simulink model "ElectronicGate"  (R2022b)
settings: Solver=VariableStepAuto  StartTime=0.0  StopTime=10.0  RelTol=1e-3
settings Model: Creator=chiar  LastModifiedBy=chiar
settings OptimizationCC: DefaultParameterBehavior=Inlined  UseDivisionForNetSlopeComputation=on  GainParamInheritBuiltInType=on  UseFloatMulNetSlope=on  InlineInvariantSignals=on  PassReuseOutputArgsAs=Individual arguments  ZeroExternalMemoryAtStartup=off  ZeroInternalMemoryAtStartup=off  NoFixptDivByZeroProtection=on  EfficientFloat2IntCast=on  LifeSpan=1  OptimizeBlockOrder=speed  DifferentSizesBufferReuse=on  EfficientTunableParamExpr=on
settings DebuggingCC: ParameterTunabilityLossMsg=error
settings HardwareCC: ProdBitPerPointer=32  ProdBitPerSizeT=32  ProdBitPerPtrDiffT=32  ProdLargestAtomicInteger=Long  ProdLargestAtomicFloat=Double  ProdWordSize=32  ProdLongLongMode=on  ProdHWDeviceType=ARM Compatible->ARM Cortex-M
settings SFSimCC: MATLABDynamicMemAlloc=off
settings RTWCC: Description=Embedded Coder  SystemTargetFile=ert.tlc  TemplateMakefile=ert_default_tmf
settings CodeAppCC: ForceParamTrailComments=on  IgnoreCustomStorageClasses=off  OperatorAnnotations=on  SimulinkDataObjDesc=on  SFDataObjDesc=on  CustomSymbolStrGlobalVar=rt$N$M  CustomSymbolStrType=$N$M  CustomSymbolStrFcn=$N$M$F  CustomSymbolStrMacro=$N$M  InsertBlockDesc=on
settings ERTTargetCC: TargetLangStandard=C99 (ISO)  GenerateSampleERTMain=on  IncludeMdlTerminateFcn=off  CombineSignalStateStructs=on  SupportComplex=off  SupportContinuousTime=on  SupportNonInlinedSFcns=on  InlinedParameterPlacement=NonHierarchical  ERTCustomFileTemplate=example_file_process.tlc  ERTFilePackagingFormat=CompactWithDataFile
settings ConfigComp: CovEnable=on  RecordCoverage=on  CovHTMLOptions=-sRT=1 -sVT=0 -aTS=1 -agT=1 -bRG=1 -bTC=1 -hTR=0 -nFC=0 -nFD=1 -scm=1 -bcm=1 -xEv=0 -xEM=0 -req=1  CovCumulativeReport=on  CovModelRefEnable=on

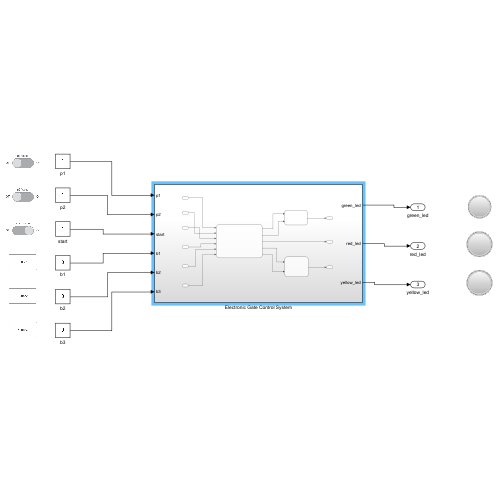
[thumbnail: Simulink's stored preview of the top-level diagram]
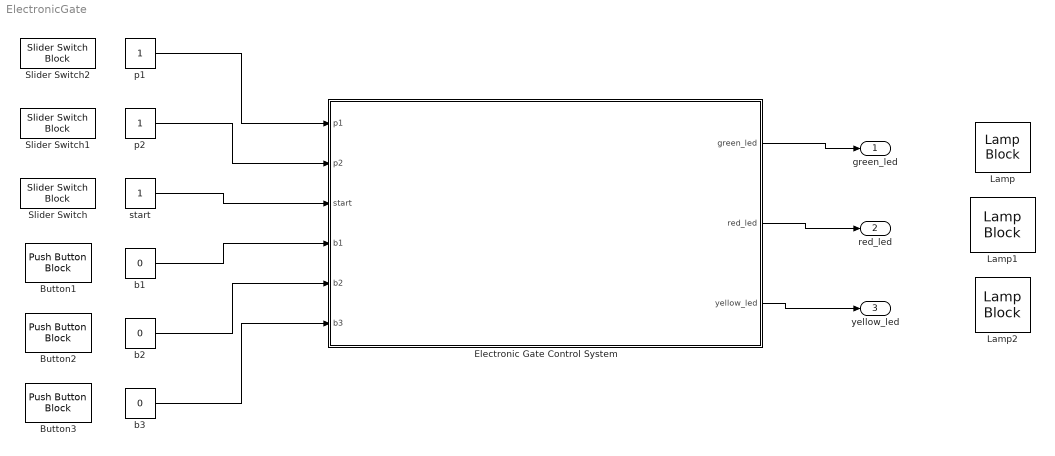
== system ElectronicGate ==
  Button1 : PushButtonBlock  ButtonText=Button1  ButtonType=Latch  OffValue=0.000000
  Button2 : PushButtonBlock  ButtonText=Button2  ButtonType=Latch  OffValue=0.000000
  Button3 : PushButtonBlock  ButtonText=Button3  ButtonType=Latch  OffValue=0.000000
  Electronic Gate Control System : Subsystem
  Lamp : LampBlock  LabelPosition=Hide
  Lamp1 : LampBlock  LabelPosition=Hide
  Lamp2 : LampBlock  LabelPosition=Hide
  Slider Switch : SliderSwitchBlock
      settings: Values={{'Off', 'On'}, [0 1]}
  Slider Switch1 : SliderSwitchBlock
      settings: Values={{'Off', 'On'}, [1 0]}
  Slider Switch2 : SliderSwitchBlock
      settings: Values={{'Off', 'On'}, [1 0]}
  b1 : Constant  Value=0  OutDataTypeStr=boolean
  b2 : Constant  Value=0  OutDataTypeStr=boolean
  b3 : Constant  Value=0  OutDataTypeStr=boolean
  p1 : Constant  OutDataTypeStr=boolean
  p2 : Constant  OutDataTypeStr=boolean
  start : Constant  OutDataTypeStr=boolean
  green_led : Outport  OutDataTypeStr=boolean
  red_led : Outport  Port=2  OutDataTypeStr=boolean
  yellow_led : Outport  Port=3  OutDataTypeStr=boolean
  wires:
  Electronic Gate Control System/1(green_led) -> green_led/1
  Electronic Gate Control System/2(red_led) -> red_led/1
  Electronic Gate Control System/3(yellow_led) -> yellow_led/1
  p1/1 -> Electronic Gate Control System/1(p1)
  p2/1 -> Electronic Gate Control System/2(p2)
  start/1 -> Electronic Gate Control System/3(start)
  b1/1 -> Electronic Gate Control System/4(b1)
  b2/1 -> Electronic Gate Control System/5(b2)
  b3/1 -> Electronic Gate Control System/6(b3)

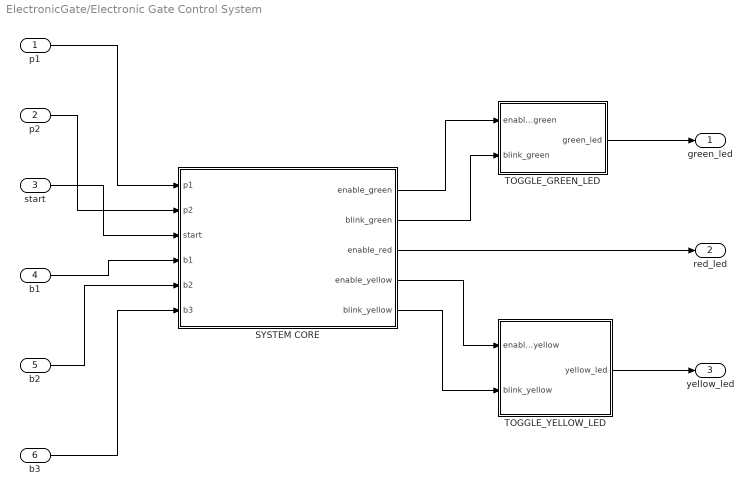
== system ElectronicGate/Electronic Gate Control System ==
  p1 : Inport  OutDataTypeStr=boolean
  p2 : Inport  Port=2  OutDataTypeStr=boolean
  start : Inport  Port=3  OutDataTypeStr=boolean
  b1 : Inport  Port=4  OutDataTypeStr=boolean
  b2 : Inport  Port=5  OutDataTypeStr=boolean
  b3 : Inport  Port=6  OutDataTypeStr=boolean
  SYSTEM CORE : Stateflow chart  TreatAsAtomicUnit=on
  TOGGLE_GREEN_LED : Stateflow chart  TreatAsAtomicUnit=on
  TOGGLE_YELLOW_LED : Stateflow chart  TreatAsAtomicUnit=on
  green_led : Outport  OutDataTypeStr=boolean
  red_led : Outport  Port=2  OutDataTypeStr=boolean
  yellow_led : Outport  Port=3  OutDataTypeStr=boolean
  wires:
  SYSTEM CORE/4(enable_yellow) -> TOGGLE_YELLOW_LED/1(enable_yellow)
  TOGGLE_YELLOW_LED/1(yellow_led) -> yellow_led/1
  p2/1 -> SYSTEM CORE/2(p2)
  start/1 -> SYSTEM CORE/3(start)
  SYSTEM CORE/5(blink_yellow) -> TOGGLE_YELLOW_LED/2(blink_yellow)
  p1/1 -> SYSTEM CORE/1(p1)
  SYSTEM CORE/1(enable_green) -> TOGGLE_GREEN_LED/1(enable_green)
  b3/1 -> SYSTEM CORE/6(b3)
  SYSTEM CORE/2(blink_green) -> TOGGLE_GREEN_LED/2(blink_green)
  b2/1 -> SYSTEM CORE/5(b2)
  SYSTEM CORE/3(enable_red) -> red_led/1
  TOGGLE_GREEN_LED/1(green_led) -> green_led/1
  b1/1 -> SYSTEM CORE/4(b1)

== stateflow chart ElectronicGate/Electronic Gate Control System/TOGGLE_GREEN_LED ==
  state TOGGLE_GREEN
    state SWITCH
      state SWITCH_OFF
        en: green_led = OFF
      state SWITCH_ON
        en: green_led = ON
      (default) -> SWITCH_OFF
      SWITCH_OFF -> SWITCH_ON : [enable_green == ON]
      SWITCH_ON -> SWITCH_OFF : [enable_green == OFF]
    state BLINKING
      state BLINKING_ON
        en: green_led = ON
      state BLINKING_OFF
        en: green_led = OFF
      (default) -> BLINKING_ON
      BLINKING_OFF -> BLINKING_ON : [after(TGREEN, sec)]
      BLINKING_ON -> BLINKING_OFF : [after(TGREEN, sec)]
    (default) -> SWITCH
    SWITCH -> BLINKING : [blink_green == ON]
    BLINKING -> SWITCH : [blink_green == OFF]
  data: TGREEN constant double =1; OFF constant boolean =0; ON constant boolean =1; enable_green input boolean; green_led output boolean; blink_green input boolean

== stateflow chart ElectronicGate/Electronic Gate Control System/SYSTEM CORE ==
  state SYSTEM
    state GATE [parallel]
      settings: executionOrder=3
      state INACTIVE
        en:
        enable_green = OFF;
        enable_yellow = OFF;
        enable_red = OFF;
        blink_green = OFF;
        blink_yellow = OFF;
      state ACTIVE
        state IS_OPENING
          en:
          enable_red = OFF;
          enable_yellow=OFF;
          enable_green=OFF;
          blink_green = OFF;
          blink_yellow = ON;
        state OPEN
          state GREEN_BLK_OFF
            en:
            enable_green = ON;
            enable_red = ON;
            enable_yellow = ON;
            blink_green = OFF;
            blink_yellow = OFF;
          state GREEN_BLK_ON
            en:
            enable_green = OFF;
            enable_red = OFF;
            enable_yellow = OFF;
            blink_green = ON;
            blink_yellow = OFF;
          (default) -> SYSTEM.GATE.ACTIVE.OPEN.GREEN_BLK_OFF
          SYSTEM.GATE.ACTIVE.OPEN.GREEN_BLK_ON -> SYSTEM.GATE.ACTIVE.OPEN.GREEN_BLK_ON [order 2] : [b1_pressed & (p1 == OFF)]
          SYSTEM.GATE.ACTIVE.OPEN.GREEN_BLK_OFF -> SYSTEM.GATE.ACTIVE.OPEN.GREEN_BLK_ON : [b1_pressed & (p1 == OFF)]
          SYSTEM.GATE.ACTIVE.OPEN.GREEN_BLK_ON -> SYSTEM.GATE.ACTIVE.OPEN.GREEN_BLK_OFF [order 1] : [after(GREENDUR, sec) | (p1 == ON)]
        state CLOSE
          state GREEN_BLK_OFF
            en:
            enable_green = OFF;
            enable_red = OFF;
            enable_yellow = OFF;
            blink_green = OFF;
            blink_yellow = OFF;
          state GREEN_BLK_ON
            en:
            enable_green = OFF;
            enable_red = OFF;
            enable_yellow = OFF;
            blink_green = ON;
            blink_yellow = OFF;
          (default) -> SYSTEM.GATE.ACTIVE.CLOSE.GREEN_BLK_OFF
          SYSTEM.GATE.ACTIVE.CLOSE.GREEN_BLK_ON -> SYSTEM.GATE.ACTIVE.CLOSE.GREEN_BLK_ON [order 2] : [b1_pressed & (p1 == OFF)]
          SYSTEM.GATE.ACTIVE.CLOSE.GREEN_BLK_OFF -> SYSTEM.GATE.ACTIVE.CLOSE.GREEN_BLK_ON : [b1_pressed & (p1 == OFF)]
          SYSTEM.GATE.ACTIVE.CLOSE.GREEN_BLK_ON -> SYSTEM.GATE.ACTIVE.CLOSE.GREEN_BLK_OFF [order 1] : [after(GREENDUR, sec) | (p1 == ON)]
        state IS_CLOSING
          en:
          enable_red = OFF;
          enable_yellow=OFF;
          enable_green=OFF;
          blink_green = OFF;
          blink_yellow = ON;
        note: Per i sensori stiamo usando la logica negata.
        state STOP_SYSTEM
          en:
          enable_red = OFF;
          enable_yellow=OFF;
          enable_green=OFF;
          blink_green = OFF;
          blink_yellow = OFF;
        state ERROR_STATE
          en:
          enable_red = ON;
          enable_yellow=OFF;
          enable_green=OFF;
          blink_green = OFF;
          blink_yellow = OFF;
        IS_OPENING -> OPEN [order 2] : after(working_time, sec)
        CLOSE -> IS_OPENING : [b1_pressed & (p1 == ON)]
        IS_CLOSING -> IS_OPENING [order 1] : [b1_pressed | (p1 == OFF)]
        IS_OPENING -> IS_CLOSING [order 1] : [b1_pressed & (p1 == ON)]
        IS_CLOSING -> CLOSE [order 2] : [(p2 == OFF)]
        (default) -> IS_CLOSING
        ERROR_STATE -> CLOSE : [p2 == OFF]
        OPEN -> IS_CLOSING : [(b1_pressed & p1 == ON) | duration(p1 == ON) >= closing_time]
        IS_CLOSING -> STOP_SYSTEM [order 3] : [after(working_time, sec) & (p2 == ON)]
        STOP_SYSTEM -> ERROR_STATE : after(WAITING_TIME,sec)
      (default) -> INACTIVE
      INACTIVE -> ACTIVE : [start == ON]
      ACTIVE -> INACTIVE : [start == OFF]
    state B1 [parallel]
      settings: executionOrder=6
      state RELEASED
      state PRESSED
      state LONG_PRESSED
        send(b1_pressed)
      (default) -> SYSTEM.B1.RELEASED
      SYSTEM.B1.RELEASED -> SYSTEM.B1.PRESSED : [b1==ON]
      SYSTEM.B1.LONG_PRESSED -> SYSTEM.B1.RELEASED : [b1 == OFF]
      SYSTEM.B1.PRESSED -> SYSTEM.B1.LONG_PRESSED : [b1 == OFF]
    state B2 [parallel]
      settings: executionOrder=5
      state RELEASED
      state PRESSED
      state LONG_PRESSED
        send(b2_pressed)
      (default) -> SYSTEM.B2.RELEASED
      SYSTEM.B2.RELEASED -> SYSTEM.B2.PRESSED : [b2==ON]
      SYSTEM.B2.LONG_PRESSED -> SYSTEM.B2.RELEASED : [b2 == OFF]
      SYSTEM.B2.PRESSED -> SYSTEM.B2.LONG_PRESSED : [b2 == OFF]
    state B3 [parallel]
      settings: executionOrder=4
      state RELEASED
      state PRESSED
      state LONG_PRESSED
        send(b3_pressed)
      (default) -> SYSTEM.B3.RELEASED
      SYSTEM.B3.RELEASED -> SYSTEM.B3.PRESSED : [b3==ON]
      SYSTEM.B3.LONG_PRESSED -> SYSTEM.B3.RELEASED : [b3 == OFF]
      SYSTEM.B3.PRESSED -> SYSTEM.B3.LONG_PRESSED : [b3 == OFF]
    state WORKING_TIME [parallel]
      settings: executionOrder=1
      state WORKING_TIME_RESET
        en:
        working_time = 10;
      state WORKING_TIME_INC
        en:
        working_time = mod(working_time, MAX) + INCREMENT;
      WORKING_TIME_INC -> WORKING_TIME_INC : [b3_pressed & p2 == OFF]
      (default) -> WORKING_TIME_RESET
      WORKING_TIME_RESET -> WORKING_TIME_INC : [b3_pressed & p2 == OFF]
    state CLOSING_TIME [parallel]
      settings: executionOrder=2
      state CLOSING_TIME_RESET
        en:
        closing_time = 10;
      state CLOSING_TIME_INC
        en:
        closing_time = mod(closing_time, MAX) + INCREMENT;
      CLOSING_TIME_INC -> CLOSING_TIME_INC : [b2_pressed & p2 == OFF]
      (default) -> CLOSING_TIME_RESET
      CLOSING_TIME_RESET -> CLOSING_TIME_INC : [b2_pressed & p2 == OFF]
  data: GREENDUR constant double =30; WAITING_TIME constant double =10; ON constant boolean =1; OFF constant boolean =0; working_time local double =10; INCREMENT constant double =10; MAX constant double =120; closing_time local double =10; p1 input boolean; p2 input boolean; start input boolean; enable_green output boolean; blink_green output boolean; enable_red output boolean; enable_yellow output boolean; blink_yellow output boolean; b1 input boolean; b2 input boolean; b3 input boolean
  events: b3_pressed local RISING_EDGE_EVENT; b1_pressed local RISING_EDGE_EVENT; b2_pressed local RISING_EDGE_EVENT

== stateflow chart ElectronicGate/Electronic Gate Control System/TOGGLE_YELLOW_LED ==
  state TOGGLE_YELLOW
    state SWITCH
      state SWITCH_OFF
        en: yellow_led = OFF
      state SWITCH_ON
        en: yellow_led = ON
      (default) -> SWITCH_OFF
      SWITCH_OFF -> SWITCH_ON : [enable_yellow == ON]
      SWITCH_ON -> SWITCH_OFF : [enable_yellow == OFF]
    state BLINKING
      state BLINKING_ON
        en: yellow_led = ON
      state BLINKING_OFF
        en: yellow_led = OFF
      (default) -> BLINKING_ON
      BLINKING_OFF -> BLINKING_ON : [after(TYELLOW, sec)]
      BLINKING_ON -> BLINKING_OFF : [after(TYELLOW, sec)]
    (default) -> SWITCH
    SWITCH -> BLINKING : [blink_yellow == ON]
    BLINKING -> SWITCH : [blink_yellow == OFF]
  data: ON constant boolean =1; OFF constant boolean =0; enable_yellow input boolean; yellow_led output boolean; TYELLOW constant double =2; blink_yellow input boolean
